simulink model "Lettura"  (R2020b)
settings: Solver=VariableStepAuto  StartTime=0.0  StopTime=10  RelTol=1e-3
values from neighbouring files (symbols this model uses):
  a = arduino('COM10', 'Due', 'Libraries', 'Serial')    [a_20210410_GPSparser.m]
undefined symbols (not defined in the file or in its folder): c, t1, val_2
libraries: svdutilitieslib x8
settings Model: Creator=lapis-dspace2  LastModifiedBy=lapis-dspace2

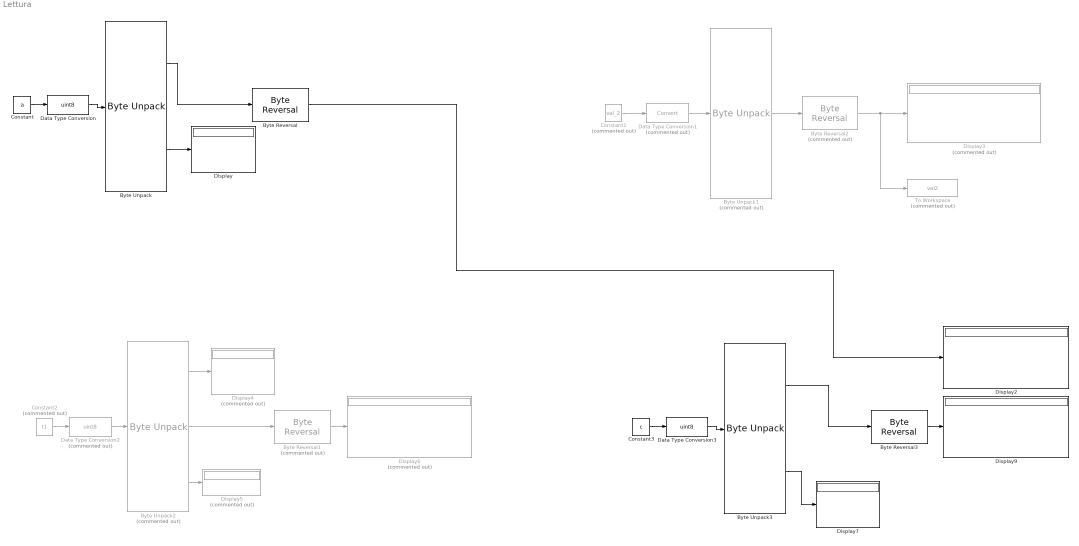
== system Lettura ==
  Byte Reversal : svdutilitieslib/Byte Reversal  numInp=1  blockPlatform=arduinoert
      settings: SourceProductBaseCode=ANDROID,ARDUINO,ML_ARDUINO,ECCORTEXA,ECCORTEXR,SC_BEAGLEBONE_BLUE,EC_FREEDOM_BOARD,EC_FRDM_K64F,INTEL_BLOCKSET,JETSONCPU,MICROBIT,NUCLEO,NVIDIA,PX4AUTOPILOTS,RASPPIIO,STMICRODIS,TIC2000,XILINX_BLOCKSET
  Byte Reversal1 : svdutilitieslib/Byte Reversal  Commented=on  numInp=1  blockPlatform=arduinoert
      settings: SourceProductBaseCode=ANDROID,ARDUINO,ML_ARDUINO,ECCORTEXA,ECCORTEXR,SC_BEAGLEBONE_BLUE,EC_FREEDOM_BOARD,EC_FRDM_K64F,INTEL_BLOCKSET,JETSONCPU,MICROBIT,NUCLEO,NVIDIA,PX4AUTOPILOTS,RASPPIIO,STMICRODIS,TIC2000,XILINX_BLOCKSET
  Byte Reversal2 : svdutilitieslib/Byte Reversal  Commented=on  numInp=1  blockPlatform=arduinoert
      settings: SourceProductBaseCode=ANDROID,ARDUINO,ML_ARDUINO,ECCORTEXA,ECCORTEXR,SC_BEAGLEBONE_BLUE,EC_FREEDOM_BOARD,EC_FRDM_K64F,INTEL_BLOCKSET,JETSONCPU,MICROBIT,NUCLEO,NVIDIA,PX4AUTOPILOTS,RASPPIIO,STMICRODIS,TIC2000,XILINX_BLOCKSET
  Byte Reversal3 : svdutilitieslib/Byte Reversal  numInp=1  blockPlatform=arduinoert
      settings: SourceProductBaseCode=ANDROID,ARDUINO,ML_ARDUINO,ECCORTEXA,ECCORTEXR,SC_BEAGLEBONE_BLUE,EC_FREEDOM_BOARD,EC_FRDM_K64F,INTEL_BLOCKSET,JETSONCPU,MICROBIT,NUCLEO,NVIDIA,PX4AUTOPILOTS,RASPPIIO,STMICRODIS,TIC2000,XILINX_BLOCKSET
  Byte Unpack : svdutilitieslib/Byte Unpack  dimensions={[12],[1]}  datatypes={'single','uint8'}  byteAlign=1  blockPlatform=arduinoert
      settings: SourceProductBaseCode=ANDROID,ARDUINO,ML_ARDUINO,ECCORTEXA,ECCORTEXR,SC_BEAGLEBONE_BLUE,EC_FREEDOM_BOARD,EC_FRDM_K64F,INTEL_BLOCKSET,JETSONCPU,MICROBIT,NUCLEO,NVIDIA,PX4AUTOPILOTS,RASPPIIO,STMICRODIS,TIC2000,XILINX_BLOCKSET
  Byte Unpack1 : svdutilitieslib/Byte Unpack  Commented=on  dimensions={[12]}  datatypes={'single'}  byteAlign=1  blockPlatform=arduinoert
      settings: SourceProductBaseCode=ANDROID,ARDUINO,ML_ARDUINO,ECCORTEXA,ECCORTEXR,SC_BEAGLEBONE_BLUE,EC_FREEDOM_BOARD,EC_FRDM_K64F,INTEL_BLOCKSET,JETSONCPU,MICROBIT,NUCLEO,NVIDIA,PX4AUTOPILOTS,RASPPIIO,STMICRODIS,TIC2000,XILINX_BLOCKSET
  Byte Unpack2 : svdutilitieslib/Byte Unpack  Commented=on  dimensions={[4],[12],[2]}  datatypes={'uint8','single','uint8'}  byteAlign=1  blockPlatform=arduinoert
      settings: SourceProductBaseCode=ANDROID,ARDUINO,ML_ARDUINO,ECCORTEXA,ECCORTEXR,SC_BEAGLEBONE_BLUE,EC_FREEDOM_BOARD,EC_FRDM_K64F,INTEL_BLOCKSET,JETSONCPU,MICROBIT,NUCLEO,NVIDIA,PX4AUTOPILOTS,RASPPIIO,STMICRODIS,TIC2000,XILINX_BLOCKSET
  Byte Unpack3 : svdutilitieslib/Byte Unpack  dimensions={[12],[1]}  datatypes={'single','uint8'}  byteAlign=1  blockPlatform=arduinoert
      settings: SourceProductBaseCode=ANDROID,ARDUINO,ML_ARDUINO,ECCORTEXA,ECCORTEXR,SC_BEAGLEBONE_BLUE,EC_FREEDOM_BOARD,EC_FRDM_K64F,INTEL_BLOCKSET,JETSONCPU,MICROBIT,NUCLEO,NVIDIA,PX4AUTOPILOTS,RASPPIIO,STMICRODIS,TIC2000,XILINX_BLOCKSET
  Constant : Constant  Value=a
  Constant1 : Constant  Commented=on  Value=val_2  OutDataTypeStr=Inherit: Inherit via back propagation
  Constant2 : Constant  Commented=on  Value=t1
  Constant3 : Constant  Value=c
  Data Type Conversion : DataTypeConversion  OutDataTypeStr=uint8
  Data Type Conversion1 : DataTypeConversion  Commented=on
  Data Type Conversion2 : DataTypeConversion  Commented=on  OutDataTypeStr=uint8
  Data Type Conversion3 : DataTypeConversion  OutDataTypeStr=uint8
  Display{,2,7,9} (4 alike) : Display
  Display{3..6} (4 alike) : Display  Commented=on
  To Workspace : ToWorkspace  Commented=on  VariableName=val2  SaveFormat=Timeseries  SampleTime=-1
  wires:
  Constant/1 -> Data Type Conversion/1
  Byte Reversal/1 -> Display2/1
  Data Type Conversion/1 -> Byte Unpack/1
  Byte Unpack1/1 -> Byte Reversal2/1
  Constant1/1 -> Data Type Conversion1/1
  Data Type Conversion1/1 -> Byte Unpack1/1
  Byte Reversal2/1 -> To Workspace/1, Display3/1
  Byte Unpack2/3 -> Display5/1
  Constant2/1 -> Data Type Conversion2/1
  Byte Unpack2/1 -> Display4/1
  Data Type Conversion2/1 -> Byte Unpack2/1
  Byte Unpack2/2 -> Byte Reversal1/1
  Byte Reversal1/1 -> Display6/1
  Constant3/1 -> Data Type Conversion3/1
  Byte Reversal3/1 -> Display9/1
  Data Type Conversion3/1 -> Byte Unpack3/1
  Byte Unpack/1 -> Byte Reversal/1
  Byte Unpack/2 -> Display/1
  Byte Unpack3/2 -> Display7/1
  Byte Unpack3/1 -> Byte Reversal3/1
